simulink model "ur10_realtime"  (R2024b)
settings: Solver=ode3  StartTime=0.0  StopTime=5  FixedStep=0.005  RelTol=1e-3
PreLoadFcn:
  | % 获取模型文件所在目录
  | modelPath = fileparts(get_param(gcs, 'FileName'));
  | 
  | % 添加相对路径
  | addpath(fullfile(modelPath, 'blocks'));
  | addpath(fullfile(modelPath, '..', 'src'));
  | 
  | % 或者使用更智能的路径查找
  | try
  |     % 尝试从当前模型位置向上查找项目根目录
  |     projectRoot = fileparts(modelPath);
  |     if contains(projectRoot, 'ur10_fault_experiments')
  |         addpath(fullfile(projectRoot, 'simulink', 'blocks'));
  |         addpath(fullfile(projectRoot, 'src'));
  |     end
  | catch
  |     % 如果失败，尝试其他方法
  |     disp('尝试其他路径设置方法...');
  | end
InitFcn:
  | % === 自动加载参数到“模型工作区” ===
  | mdl = bdroot;
  | mw  = get_param(mdl,'ModelWorkspace');
  | 
  | % 组相对路径：<模型所在目录>\blocks\params_norm.mat
  | mdlDir  = fileparts(get_param(mdl,'FileName'));
  | matFile = fullfile(mdlDir,'blocks','params_norm.mat');
  | 
  | S = load(matFile);  % 期望里面有 S.xmin_pose / S.xmax_pose
  | 
  | % 将变量写入模型工作区（而非 base workspace，避免污染）
  | mw.assignin('xmin_pose', S.normp.xmin);
  | mw.assignin('xmax_pose', S.normp.xmax);
model workspace (MAT data in the model file):
  xmax_pose = [-185.008835287 -256.096489307 623.604405501 90.0021784312 0 0.5]
  xmin_pose = [-576.609188137 -385.089682718 463.733604749 76.7568601853 -14.5267505859 -5.92723883093]
settings Model: Creator=Jinch  LastModifiedBy=Jinch

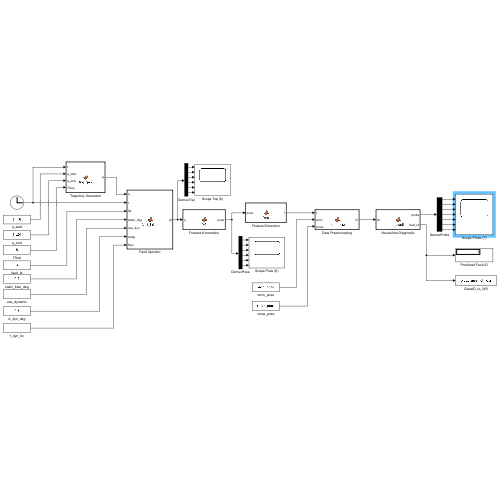
[thumbnail: Simulink's stored preview of the top-level diagram]
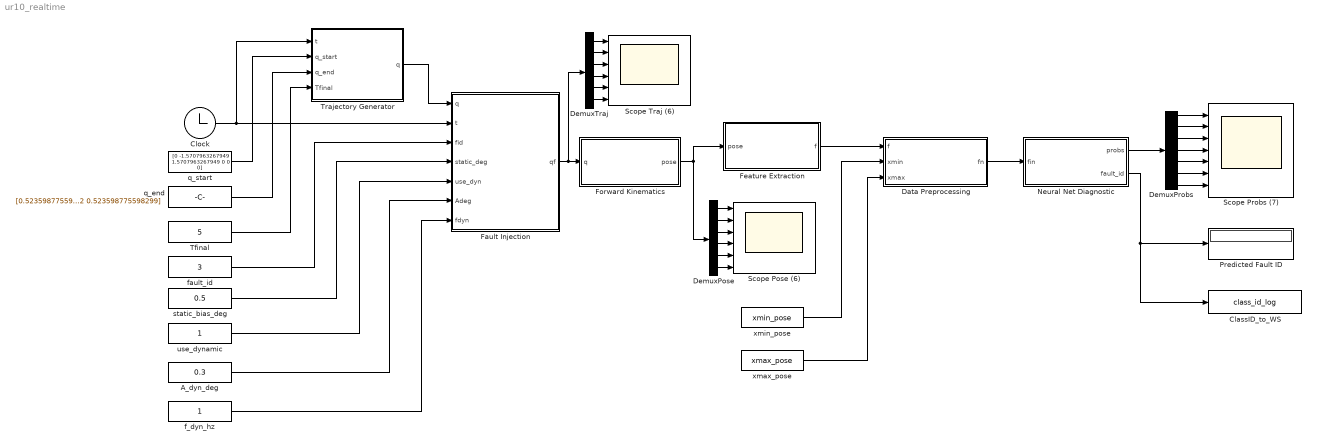
== system ur10_realtime ==
  A_dyn_deg : Constant  Value=0.3
  ClassID_to_WS : ToWorkspace  VariableName=class_id_log  SampleTime=-1
  Clock : Clock
  Data Preprocessing : MATLAB Function  TreatAsAtomicUnit=on
  DemuxPose : Demux  Outputs=6
  DemuxProbs : Demux  Outputs=7
  DemuxTraj : Demux  Outputs=6
  Fault Injection : MATLAB Function  TreatAsAtomicUnit=on
  Feature Extraction : MATLAB Function  TreatAsAtomicUnit=on
  Forward Kinematics : MATLAB Function  TreatAsAtomicUnit=on
  Neural Net Diagnostic : MATLAB Function  TreatAsAtomicUnit=on
  Predicted Fault ID : Display
  Scope Pose (6) : Scope  NumInputPorts=6
  Scope Probs (7) : Scope  NumInputPorts=7
  Scope Traj (6) : Scope  NumInputPorts=6
  Tfinal : Constant  Value=5
  Trajectory Generator : MATLAB Function  TreatAsAtomicUnit=on
  f_dyn_hz : Constant
  fault_id : Constant  Value=3
  q_end : Constant  Value=[0.523598775598299 -2.0943951023932 2.26892802759263 -0.523598775598299 0.698131700797732 0.523598775598299]
  q_start : Constant  Value=[0 -1.5707963267949 1.5707963267949 0 0 0]
  static_bias_deg : Constant  Value=0.5
  use_dynamic : Constant
  xmax_pose : Constant  Value=xmax_pose
  xmin_pose : Constant  Value=xmin_pose
  wires:
  Clock/1 -> Trajectory Generator/1(t), Fault Injection/2(t)
  q_start/1 -> Trajectory Generator/2(q_start)
  q_end/1 -> Trajectory Generator/3(q_end)
  Tfinal/1 -> Trajectory Generator/4(Tfinal)
  fault_id/1 -> Fault Injection/3(fid)
  static_bias_deg/1 -> Fault Injection/4(static_deg)
  use_dynamic/1 -> Fault Injection/5(use_dyn)
  A_dyn_deg/1 -> Fault Injection/6(Adeg)
  f_dyn_hz/1 -> Fault Injection/7(fdyn)
  Fault Injection/1(qf) -> DemuxTraj/1, Forward Kinematics/1(q)
  Forward Kinematics/1(pose) -> Feature Extraction/1(pose), DemuxPose/1
  Feature Extraction/1(f) -> Data Preprocessing/1(f)
  xmin_pose/1 -> Data Preprocessing/2(xmin)
  xmax_pose/1 -> Data Preprocessing/3(xmax)
  Data Preprocessing/1(fn) -> Neural Net Diagnostic/1(fin)
  DemuxPose/1 -> Scope Pose (6)/1
  DemuxPose/2 -> Scope Pose (6)/2
  DemuxPose/3 -> Scope Pose (6)/3
  DemuxPose/4 -> Scope Pose (6)/4
  DemuxPose/5 -> Scope Pose (6)/5
  DemuxPose/6 -> Scope Pose (6)/6
  Neural Net Diagnostic/1(probs) -> DemuxProbs/1
  DemuxProbs/1 -> Scope Probs (7)/1
  DemuxProbs/2 -> Scope Probs (7)/2
  DemuxProbs/3 -> Scope Probs (7)/3
  DemuxProbs/4 -> Scope Probs (7)/4
  DemuxProbs/5 -> Scope Probs (7)/5
  DemuxProbs/6 -> Scope Probs (7)/6
  DemuxProbs/7 -> Scope Probs (7)/7
  Neural Net Diagnostic/2(fault_id) -> Predicted Fault ID/1, ClassID_to_WS/1
  DemuxTraj/2 -> Scope Traj (6)/2
  DemuxTraj/3 -> Scope Traj (6)/3
  DemuxTraj/5 -> Scope Traj (6)/5
  DemuxTraj/4 -> Scope Traj (6)/4
  DemuxTraj/6 -> Scope Traj (6)/6
  Trajectory Generator/1(q) -> Fault Injection/1(q)
  DemuxTraj/1 -> Scope Traj (6)/1

== matlab function ur10_realtime/Fault Injection ==
  data: q input; qf output; t input; fid input; static_deg input; use_dyn input; Adeg input; fdyn input
function qf = fault_inject(q, t, fid, static_deg, use_dyn, Adeg, fdyn)

d2r = pi/180;
qf = q(:);
if fid > 0 && fid <= 6
  qf(fid) = qf(fid) + static_deg*d2r;
  if use_dyn ~= 0
    qf(fid) = qf(fid) + (Adeg*d2r)*sin(2*pi*fdyn*t);
  end
end

end

== matlab function ur10_realtime/Trajectory Generator ==
  data: t input; q output; q_start input; q_end input; Tfinal input
function q = traj_gen(t, q_start, q_end, Tfinal)
% 线性插值轨迹生成器
% 输入: t - 当前时间
%       q_start - 起始位置向量
%       q_end - 目标位置向量
%       Tfinal - 总运动时间
% 输出: q - 当前位置向量

q = zeros(6,1);
qs = q_start(:); qe = q_end(:);

if t <= 0
  q = qs;              % 时间小于等于0，返回起始位置
elseif t >= Tfinal
  q = qe;              % 时间大于等于总时间，返回目标位置
else
  % 线性插值
  tau = t / Tfinal;    % 归一化时间参数 [0,1]
  q = qs + tau * (qe - qs);  % 线性插值公式

  % s  = (10*tau^3 - 15*tau^4 + 6*tau^5);   % 五次多项式差值
  % q  = qs + s*(qe - qs);

end
end

== matlab function ur10_realtime/Forward Kinematics ==
  data: q input; pose output
function pose = fk6(q)
%#codegen
pose = zeros(1,6);
coder.extrinsic('fwd_kinematics_ur10','euler_zyx_from_R');

q_deg = q * 180/pi;
T06 = fwd_kinematics_ur10(q_deg);
R = zeros(3,3); 
p = zeros(1,3);
if ~isempty(T06)
  R = T06(1:3,1:3);
  p = T06(1:3,4)';
end
eul = zeros(1,3);
if ~isempty(R)
  eul = euler_zyx_from_R(R);
end
pose = [p, eul];

end

== matlab function ur10_realtime/Feature Extraction ==
  data: pose input; f output
function f = feat(pose)
%#codegen
if isequal(size(pose),[6 1])
  f = pose';
else
  f = reshape(pose,1,6);
end
end

== matlab function ur10_realtime/Data Preprocessing ==
  data: f input; fn output; xmin input; xmax input
function fn = preprocess(f, xmin, xmax)
%#codegen
f    = reshape(f,1,6);
xmin = reshape(xmin,1,6);
xmax = reshape(xmax,1,6);
epsv = 1e-9;
fn   = (f - xmin) ./ max(xmax - xmin, epsv);
end

== matlab function ur10_realtime/Neural Net Diagnostic ==
  data: fin input; probs output; fault_id output
function [probs, fault_id] = nn_predict(fin)
%#codegen
% 恒定输出：probs 1x7(double)，class_id 1x1(int32)

probs    = zeros(1,7);   % 预分配固定尺寸
fault_id = int32(0);

% 将输入组织为“列为样本”的 6x1
x = reshape(fin, 6, 1);

% 声明外部函数并用“固定形状的接收变量”接住返回值
coder.extrinsic('predict_bpn');
y = zeros(7,1);          % 期望网络返回 7x1（Q=1）
y = predict_bpn(x);      % 直接赋值给已定型的 double 变量

% 现在 y 已是 double(7x1)，可以安全运算
probs = y.';             % 转成 1x7
[~, k] = max(probs, [], 2);
fault_id = int32(k)-1;
end
